simulink model "mahony_alg"  (R2018a)
settings: Solver=FixedStepAuto  StartTime=0.0  StopTime=inf  FixedStep=0.01  RelTol=1e-3  EnableMultiTasking=on
InitFcn:
  | set_param('step_test/Output/Run Sim','Value','1');
  | set_param('step_test/Motor Switch','Value','0');
  | set_param('step_test/Automatic Control','Value','0');
  | %set_param('step_test/Manual PWM','Gain','0');
undefined symbols (not defined in the file or in its folder): sigbuilder_block
libraries: simulink x4, arduinolib x3, dspstat3 x1, dspfdesign x1
settings Model: SimulationMode=external  ExtModeTrigDuration=2  Creator=adiravishankara  LastModifiedBy=adiravishankara
settings SolverCC: AutoInsertRateTranBlk=on
settings OptimizationCC: EnhancedBackFolding=on  PassReuseOutputArgsThreshold=0  MaxStackSize=64  OptimizeBlockOrder=speed  DifferentSizesBufferReuse=on  OptimizationCustomize=off
settings DebuggingCC: ParameterTunabilityLossMsg=error
settings HardwareCC: ProdBitPerPointer=32  ProdBitPerSizeT=32  ProdBitPerPtrDiffT=32  ProdLargestAtomicInteger=Long  ProdLargestAtomicFloat=Double  ProdWordSize=32  ProdHWDeviceType=ARM Compatible->ARM Cortex  UseEmbeddedCoderFeatures=off
settings SFSimCC: MATLABDynamicMemAlloc=off
settings RTWCC: SystemTargetFile=ert.tlc  HardwareBoard=Arduino Due  TLCOptions=-aInlineSetEventsForThisBaseRateFcn=TLC_FALSE -aSuppressMultiTaskScheduler=TLC_FALSE -aRateBasedStepFcn=1  TemplateMakefile=ert_default_tmf  GenerateReport=on  Toolchain=Arduino ARM  BuildConfiguration=Faster Runs  LaunchReport=on
settings CodeAppCC: ForceParamTrailComments=on  OperatorAnnotations=on
settings ERTTargetCC: ERTCustomFileBanners=off  SupportContinuousTime=on  SupportNonInlinedSFcns=on  RemoveResetFunc=off  SupportVariableSizeSignals=on  ModelStepFunctionPrototypeControlCompliant=off

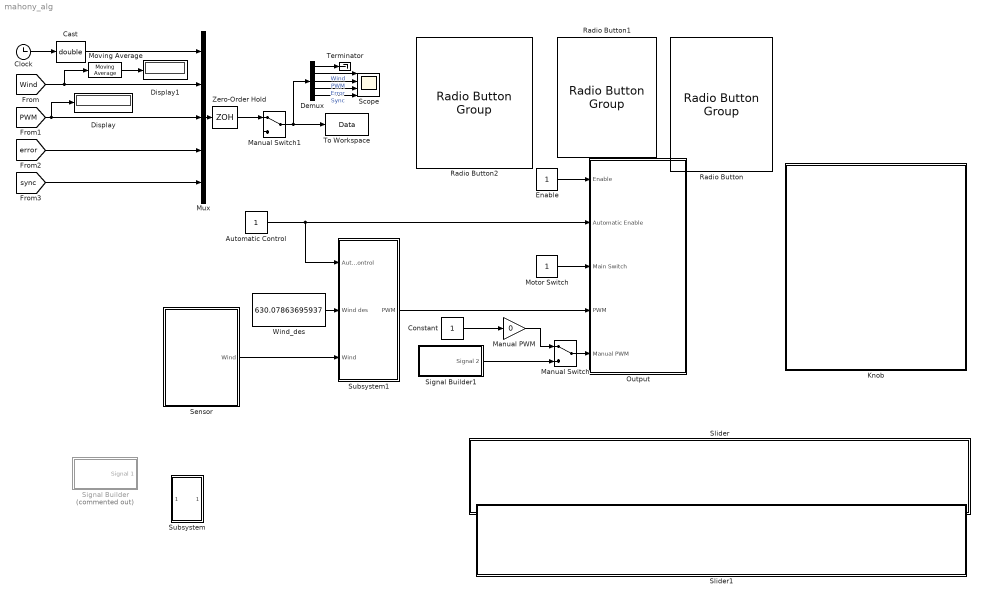
== system mahony_alg ==
  Automatic Control : Constant  SampleTime=0.01
  Cast : DataTypeConversion  OutDataTypeStr=double
  Clock : Clock
  Constant : Constant  SampleTime=0.01
  Demux : Demux  Outputs=5
  Display : Display
  Display1 : Display
  Enable : Constant  SampleTime=0.01
  Knob : Subsystem  DialogController=hmiCreateDDGDialog  IsWebBlock=on  mask(MWDashboardBlock){webBlockId=852d3d9e-f600-4180-8955-96c4171a0510, webBlockType=continuousknob, ShowInLibBrowser=on, ShowInitialText=on, HMISrcModelName=mahony_alg}
      mask prompts: webBlockId "WebBlock Id"; webBlockType "WebBlock Type"; HMISrcModelName "Source Model"
      mask help: SimulinkHMI:dialogs:ContinuousKnobDialogDesc
      mask Help: helpview([docroot '/mapfiles/simulink.map'], 'hmi_knob')
      mask Display:
      | if strcmp(get_param(bdroot(gcb),'BlockDiagramType'), 'library')
      |     image([(matlabroot) '/toolbox/simulink/hmi/icons/ContinuousKnob.png']);
      | end
  Manual PWM : Gain  Gain=0
  Manual Switch : ManualSwitch
  Manual Switch1 : ManualSwitch
  Motor Switch : Constant  SampleTime=0.01
  Moving Average : dspstat3/Moving Average  Method=Sliding window  ForgettingFactorPort=off  SpecifyWindowLength=on  WindowLength=5  ForgettingFactor=0.9  SimulateUsing=Code generation
  Mux : Mux  Inputs=5
  Output : Subsystem
  Radio Button : RadioButtonGroup  WebBlockId=124  SelectedLabel=OFF  ButtonGroupName=SIM STATUS
      settings: Values={{'ON', 'OFF'}, [1 0]}
  Radio Button1 : RadioButtonGroup  WebBlockId=141  SelectedLabel=ON  ButtonGroupName=SIM STATUS
      settings: Values={{'ON', 'OFF'}, [1 0]}
  Radio Button2 : RadioButtonGroup  WebBlockId=144  SelectedLabel=ON  ButtonGroupName=SIM STATUS
      settings: Values={{'ON', 'OFF'}, [1 0]}
  Scope : Scope  NumInputPorts=4
  Sensor : Subsystem
  Signal Builder : Subsystem  Tag=STV Subsys  Commented=on  LoadFcn=sigbuilder_block('load');  StartFcn=sigbuilder_block('start');  StopFcn=sigbuilder_block('stop');  ClipboardFcn=sigbuilder_block('clipboard');  mask(Sigbuilder block){tuvar=[0:10]}
      mask help: Simulink:masks:SigbuilderBlock_MD
      mask init:
      | if ~strcmp(get_param(bdroot(gcbh),'SimulationStatus'),'stopped') tuvar = sigbuilder_block('maskInit'); end
      settings: CopyFcn=sigbuilder_block('copy');  DeleteFcn=sigbuilder_block('delete');  ModelCloseFcn=sigbuilder_block('modelClose');  PreSaveFcn=sigbuilder_block('preSave');  PauseFcn=sigbuilder_block('pause');  ContinueFcn=sigbuilder_block('continue');  NameChangeFcn=sigbuilder_block('namechange');  OpenFcn=sigbuilder_block('open',[48.75 0 1391.25 729.75 ]);  CloseFcn=sigbuilder_block('close');
      mask Display: plot(0, 0, 100, 100,[2, 2, 32, 32, 2], [68, 8, 8, 68, 68],[32, 2], [38, 38], [32, 19, 2],[53, 60, 44], [32, 17, 17, 2],[16, 16, 31, 31]);txt = getActiveGroup(gcbh);text(2, 100, txt,'verticalAlignment', 'top');
  Signal Builder1 : Subsystem  Tag=STV Subsys  LoadFcn=sigbuilder_block('load');  StartFcn=sigbuilder_block('start');  StopFcn=sigbuilder_block('stop');  ClipboardFcn=sigbuilder_block('clipboard');  mask(Sigbuilder block){tuvar=[0:10]}
      mask help: Simulink:masks:SigbuilderBlock_MD
      mask init:
      | if ~strcmp(get_param(bdroot(gcbh),'SimulationStatus'),'stopped') tuvar = sigbuilder_block('maskInit'); end
      settings: CopyFcn=sigbuilder_block('copy');  DeleteFcn=sigbuilder_block('delete');  ModelCloseFcn=sigbuilder_block('modelClose');  PreSaveFcn=sigbuilder_block('preSave');  PauseFcn=sigbuilder_block('pause');  ContinueFcn=sigbuilder_block('continue');  NameChangeFcn=sigbuilder_block('namechange');  OpenFcn=sigbuilder_block('open',[48.75 0 1391.25 711 ]);  CloseFcn=sigbuilder_block('close');
      mask Display: plot(0, 0, 100, 100,[2, 2, 32, 32, 2], [68, 8, 8, 68, 68],[32, 2], [38, 38], [32, 19, 2],[53, 60, 44], [32, 17, 17, 2],[16, 16, 31, 31]);txt = getActiveGroup(gcbh);text(2, 100, txt,'verticalAlignment', 'top');
  Slider : Subsystem  DialogController=hmiCreateDDGDialog  IsWebBlock=on  mask(MWDashboardBlock){webBlockId=6d6bce73-9061-4720-a103-f9820fa904f8, webBlockType=slider, ShowInLibBrowser=on, ShowInitialText=on, HMISrcModelName=mahony_alg}
      mask prompts: webBlockId "WebBlock Id"; webBlockType "WebBlock Type"; HMISrcModelName "Source Model"
      mask help: SimulinkHMI:dialogs:SliderDialogDesc
      mask Help: helpview([docroot '/mapfiles/simulink.map'], 'hmi_slider')
      mask Display:
      | if strcmp(get_param(bdroot(gcb),'BlockDiagramType'), 'library')
      |     image([(matlabroot) '/toolbox/simulink/hmi/icons/Slider.png']);
      | end
  Slider1 : Subsystem  DialogController=hmiCreateDDGDialog  IsWebBlock=on  mask(MWDashboardBlock){webBlockId=583235cf-a666-476d-a93b-c374fcd1b609, webBlockType=slider, ShowInLibBrowser=on, ShowInitialText=on, HMISrcModelName=mahony_alg}
      mask prompts: webBlockId "WebBlock Id"; webBlockType "WebBlock Type"; HMISrcModelName "Source Model"
      mask help: SimulinkHMI:dialogs:SliderDialogDesc
      mask Help: helpview([docroot '/mapfiles/simulink.map'], 'hmi_slider')
      mask Display:
      | if strcmp(get_param(bdroot(gcb),'BlockDiagramType'), 'library')
      |     image([(matlabroot) '/toolbox/simulink/hmi/icons/Slider.png']);
      | end
  Subsystem : Subsystem
  Subsystem1 : Subsystem
  Terminator : Terminator
  To Workspace : ToWorkspace  VariableName=Data  SampleTime=-1
      settings: Save2DSignal=2-D array (concatenate along first dimension)
  Wind_des : Constant  Value=630.07863695937  SampleTime=0.01
  Zero-Order Hold : ZeroOrderHold  SampleTime=0.01
  wires:
  Manual PWM/1 -> Manual Switch/1
  Motor Switch/1 -> Output/3(Main Switch)
  Enable/1 -> Output/1(Enable)
  Constant/1 -> Manual PWM/1
  Wind_des/1 -> Subsystem1/2(Wind des)
  Subsystem1/1(PWM) -> Output/4(PWM)
  Automatic Control/1 -> Subsystem1/1(Automatic Control), Output/2(Automatic Enable)
  Sensor/1(Wind) -> Subsystem1/3(Wind)
  Mux/1 -> Zero-Order Hold/1
  [Wind] -> Mux/2, Moving Average/1
  [PWM] -> Mux/3, Display/1
  [error] -> Mux/4
  Clock/1 -> Cast/1
  Cast/1 -> Mux/1
  [sync] -> Mux/5
  Manual Switch/1 -> Output/5(Manual PWM)
  Moving Average/1 -> Display1/1
  Signal Builder1/1(Signal 2) -> Manual Switch/2
  Manual Switch1/1 -> Demux/1, To Workspace/1
  Zero-Order Hold/1 -> Manual Switch1/1
  Demux/2 -> Scope/1  "Wind"
  Demux/5 -> Scope/4  "Sync"
  Demux/4 -> Scope/3  "Error"
  Demux/3 -> Scope/2  "PWM"
  Demux/1 -> Terminator/1

== system mahony_alg/Knob ==

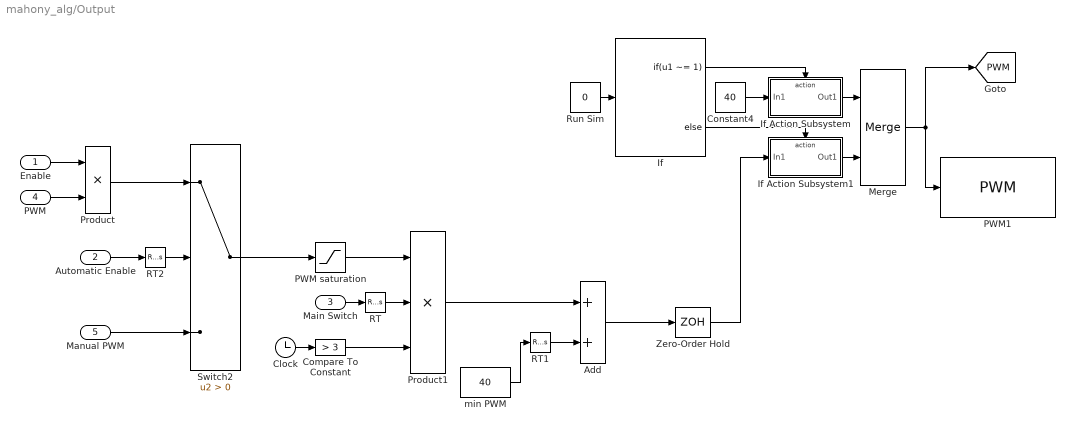
== system mahony_alg/Output ==
  Enable : Inport
  Automatic Enable : Inport  Port=2
  Main Switch : Inport  Port=3
  PWM : Inport  Port=4
  Manual PWM : Inport  Port=5
  Add : Sum
  Clock : Clock
      settings: Decimation=2
  Compare To Constant : simulink/Logic and Bit Operations/Compare To Constant  relop=>  const=3  OutDataTypeStr=boolean
  Constant4 : Constant  Value=40  SampleTime=0.01
  If : If  IfExpression=u1 ~= 1
  If Action Subsystem : Subsystem  TreatAsAtomicUnit=on
  If Action Subsystem1 : Subsystem  TreatAsAtomicUnit=on
  Merge : Merge
  PWM saturation : Saturate  UpperLimit=40  LowerLimit=0
  PWM1 : arduinolib/PWM  pinNumber=12  EnableInputFrequency=off  InitialFrequency=2000  InitialDutyCycle=0  NotificationType=None  blockPlatform=arduino
  Product : Product
  Product1 : Product  Inputs=3
  RT : RateTransition  OutPortSampleTime=0.01
  RT1 : RateTransition  OutPortSampleTime=0.01
  RT2 : RateTransition  OutPortSampleTime=0.01
  Run Sim : Constant  Value=0  SampleTime=0.01
  Switch2 : Switch  Criteria=u2 > Threshold
  Zero-Order Hold : ZeroOrderHold  SampleTime=0.01
  min PWM : Constant  Value=40  SampleTime=0.01
  tag scope: PWM=global
  wires:
  Clock/1 -> Compare To Constant/1
  min PWM/1 -> RT1/1
  Compare To Constant/1 -> Product1/3
  Automatic Enable/1 -> RT2/1
  Manual PWM/1 -> Switch2/3
  PWM/1 -> Product/2
  Switch2/1 -> PWM saturation/1
  Main Switch/1 -> RT/1
  Product1/1 -> Add/1
  PWM saturation/1 -> Product1/1
  Product/1 -> Switch2/1
  Enable/1 -> Product/1
  If/1 -> If Action Subsystem/Action
  Run Sim/1 -> If/1
  Constant4/1 -> If Action Subsystem/1(In1)
  Add/1 -> Zero-Order Hold/1
  If/2 -> If Action Subsystem1/Action
  If Action Subsystem/1(Out1) -> Merge/1
  If Action Subsystem1/1(Out1) -> Merge/2
  Merge/1 -> PWM1/1, [PWM]
  Zero-Order Hold/1 -> If Action Subsystem1/1(In1)
  RT/1 -> Product1/2
  RT1/1 -> Add/2
  RT2/1 -> Switch2/2

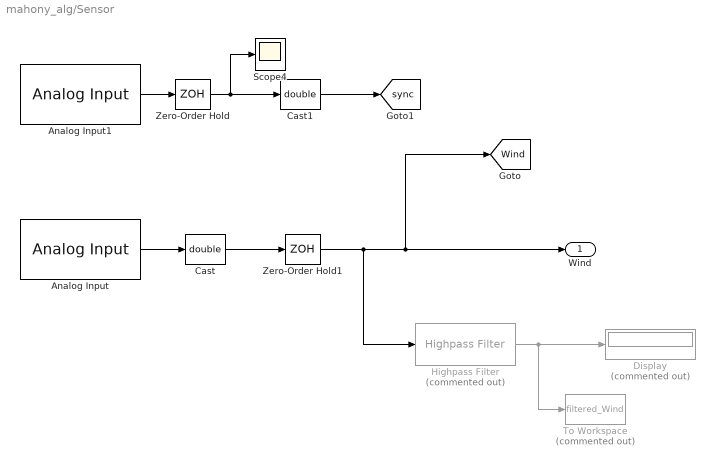
== system mahony_alg/Sensor ==
  Analog Input : arduinolib/Analog Input  pinNumber=2  ReadResultsOnly=off  ConversionTriggerSource=Software  ExternalTriggerType=uint32(0)  OutputDataType=uint16  EnableConversionCompleteNotify=off  EnableOuputStatus=off  SampleTime=0.01  blockPlatform=arduino
  Analog Input1 : arduinolib/Analog Input  pinNumber=3  ReadResultsOnly=off  ConversionTriggerSource=Software  ExternalTriggerType=uint32(0)  OutputDataType=uint16  EnableConversionCompleteNotify=off  EnableOuputStatus=off  SampleTime=0.01  blockPlatform=arduino
  Cast : DataTypeConversion  OutDataTypeStr=double
  Cast1 : DataTypeConversion  OutDataTypeStr=double
  Display : Display  Commented=on
  Highpass Filter : dspfdesign/Highpass Filter  Commented=on  FilterType=FIR  DesignForMinimumOrder=on  FilterOrder=50  StopbandFrequency=8e3  PassbandFrequency=12e3  StopbandAttenuation=80  PassbandRipple=0.1  InheritSampleRate=on  SampleRate=44100  SimulateUsing=Interpreted execution  roundingMode=Floor  coeffsDataTypeStr=fixdt(1,16)
      settings: SourceProductName=DSP System Toolbox
  Scope4 : Scope
  To Workspace : ToWorkspace  Commented=on  VariableName=filtered_Wind  SampleTime=0.01
  Zero-Order Hold : ZeroOrderHold  SampleTime=0.01
  Zero-Order Hold1 : ZeroOrderHold  SampleTime=0.01
  Wind : Outport
  tag scope: Wind=global, sync=global
  wires:
  Zero-Order Hold/1 -> Cast1/1, Scope4/1
  Analog Input/1 -> Cast/1
  Cast/1 -> Zero-Order Hold1/1
  Analog Input1/1 -> Zero-Order Hold/1
  Cast1/1 -> [sync]
  Zero-Order Hold1/1 -> Highpass Filter/1, Wind/1, [Wind]
  Highpass Filter/1 -> To Workspace/1, Display/1

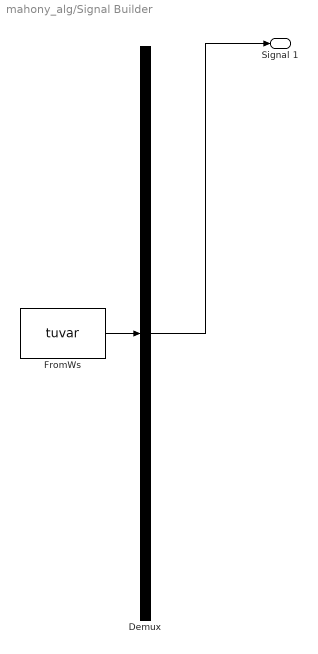
== system mahony_alg/Signal Builder ==
  Demux : Demux  Tag=STV Demux  Outputs=1
  FromWs : FromWorkspace  Tag=STV FromWs  VariableName=tuvar  SampleTime=0
      SigBuilderData=|
      | common.afterFinalStr = 'Extrapolate'
      | common.sampleTime = 0
      | dataSet.timeRange = [0 500]
      | dataSet.name = 'Group 1'
      | sbobj.Groups.Name = 'Group 1'
      | sbobj.Groups.Signals.Name = 'Signal 1'
      | sbobj.Groups.Signals.XData = [0 10 10 30 30 50 50 70 70 90 90 110 110 130 130 150 150 170 170 190 190 210 210 230 230 250 250 270 270 289 290 310 310 330 330 350 350 370 370 390 390 410 410 450 450 500]
      | sbobj.Groups.Signals.YData = [0 0 4 4 4.1 4.1 4.2 4.2 4.3 4.3 4.4 4.4 4.5 4.5 4.6 4.6 4.7 4.7 4.8 4.8 4.9 4.9 5 5 5.1 5.1 5.2 5.2 5.3 5.3 5.4 5.4 5.5 5.5 5.6 5.6 5.7 5.7 5.8 5.8 5.9 5.9 6 6 0 0]
      | sbobj.Groups.TimeRange = [0 500]
  Signal 1 : Outport  Tag=STV Outport
  wires:
  Demux/1 -> Signal 1/1
  FromWs/1 -> Demux/1

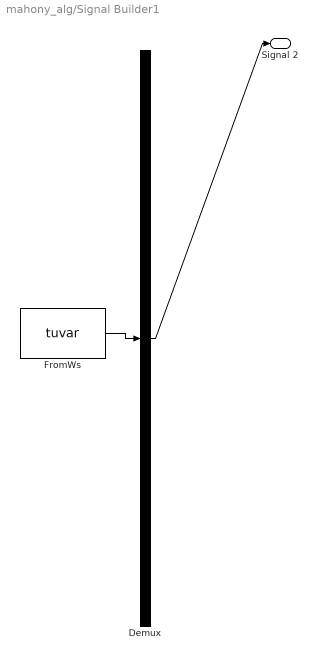
== system mahony_alg/Signal Builder1 ==
  Demux : Demux  Tag=STV Demux  Outputs=1
  FromWs : FromWorkspace  Tag=STV FromWs  VariableName=tuvar  SampleTime=0
      SigBuilderData=|
      | common.afterFinalStr = 'Extrapolate'
      | common.sampleTime = 0
      | dataSet.timeRange = [0 300]
      | dataSet.name = 'Group 1'
      | sbobj.Groups.Name = 'Group 1'
      | sbobj.Groups.Signals.Name = 'Signal 2'
      | sbobj.Groups.Signals.XData = [0 60 60 119 119 179 179 239 239 299 299 300]
      | sbobj.Groups.Signals.YData = [0 0 4 4 5 5 6 6 7 7 8 8]
      | sbobj.Groups.TimeRange = [0 300]
  Signal 2 : Outport  Tag=STV Outport
  wires:
  FromWs/1 -> Demux/1
  Demux/1 -> Signal 2/1

== system mahony_alg/Slider ==

== system mahony_alg/Slider1 ==

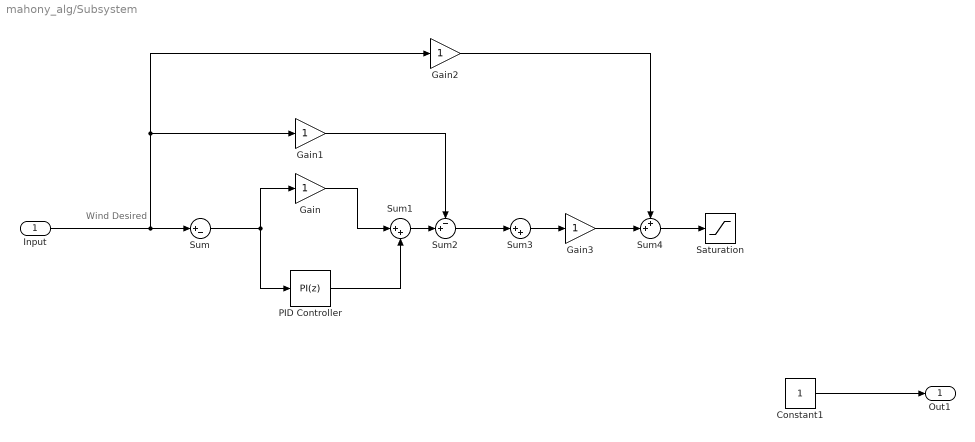
== system mahony_alg/Subsystem ==
  note: Wind Desired
  Input : Inport
  Constant1 : Constant
  Gain{,1..3} (4 alike) : Gain
  PID Controller : simulink/Continuous/PID Controller  Controller=PI  TimeDomain=Discrete-time  SampleTime=-1  IntegratorMethod=Forward Euler  FilterMethod=Forward Euler  Form=Parallel  UseFilter=on  ControllerParametersSource=internal  P=1  I=1  D=0  N=100  InitialConditionSource=internal  InitialConditionForIntegrator=0  InitialConditionForFilter=0  ExternalReset=none  LimitOutput=off  UpperSaturationLimit=inf  LowerSaturationLimit=-inf  LinearizeAsGain=on  AntiWindupMode=none  Kb=1  TrackingMode=off  Kt=1  PParamMin=[]  PParamMax=[]  IParamMin=[]  IParamMax=[]  DParamMin=[]  DParamMax=[]  NParamMin=[]  NParamMax=[]  KbParamMin=[]  KbParamMax=[]  KtParamMin=[]  KtParamMax=[]  POutMin=[]  POutMax=[]  IOutMin=[]  IOutMax=[]  DOutMin=[]  DOutMax=[]  NOutMin=[]  NOutMax=[]  KbOutMin=[]  KbOutMax=[]  KtOutMin=[]  KtOutMax=[]  IntegratorOutMin=[]  IntegratorOutMax=[]  FilterOutMin=[]  FilterOutMax=[]  SumOutMin=[]  SumOutMax=[]  SumI1OutMin=[]  SumI1OutMax=[]  SumI2OutMin=[]  SumI2OutMax=[]  SumI3OutMin=[]  SumI3OutMax=[]  SumDOutMin=[]  SumDOutMax=[]  SaturationOutMin=[]  SaturationOutMax=[]  IntegratorContinuousStateAttributes=''  IntegratorStateMustResolveToSignalObject=off  IntegratorRTWStateStorageClass=Auto  FilterContinuousStateAttributes=''  FilterStateMustResolveToSignalObject=off  FilterRTWStateStorageClass=Auto  DifferentiatorICPrevScaledInput=0  DifferentiatorOutMin=[]  DifferentiatorOutMax=[]  InitialConditionSetting=Output  FilterDiffOutCoefMin=[]  FilterDiffOutCoefMax=[]  SumDenOutMin=[]  SumDenOutMax=[]  SumNumOutMin=[]  SumNumOutMax=[]  ReciprocalOutMin=[]  ReciprocalOutMax=[]  DivideOutMin=[]  DivideOutMax=[]  TunerSelectOption=Transfer Function Based (PID Tuner App)
  Saturation : Saturate
  Sum : Sum  Inputs=|+-
  Sum1 : Sum  Inputs=|++
  Sum2 : Sum  Inputs=-+|
  Sum3 : Sum  Inputs=|++
  Sum4 : Sum  Inputs=++|
  Out1 : Outport
  wires:
  Constant1/1 -> Out1/1
  Input/1 -> Sum/1, Gain2/1, Gain1/1
  Sum/1 -> PID Controller/1, Gain/1
  Gain/1 -> Sum1/1
  PID Controller/1 -> Sum1/2
  Sum1/1 -> Sum2/2
  Gain1/1 -> Sum2/1
  Sum2/1 -> Sum3/1
  Sum3/1 -> Gain3/1
  Gain3/1 -> Sum4/2
  Gain2/1 -> Sum4/1
  Sum4/1 -> Saturation/1

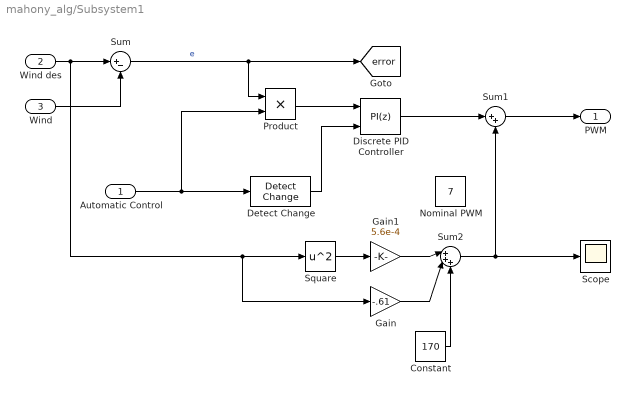
== system mahony_alg/Subsystem1 ==
  Automatic Control : Inport
  Wind des : Inport  Port=2
  Wind : Inport  Port=3
  Constant : Constant  Value=170
  Detect Change : simulink/Logic and Bit Operations/Detect Change  vinit=0  OutDataTypeStr=boolean
  Discrete PID Controller : simulink/Continuous/PID Controller  Controller=PI  TimeDomain=Discrete-time  SampleTime=0.01  IntegratorMethod=Forward Euler  FilterMethod=Forward Euler  Form=Parallel  UseFilter=on  ControllerParametersSource=internal  P=0.05  I=0.01  D=0  N=100  InitialConditionSource=internal  InitialConditionForIntegrator=0  InitialConditionForFilter=0  ExternalReset=rising  LimitOutput=off  UpperSaturationLimit=inf  LowerSaturationLimit=-inf  LinearizeAsGain=off  AntiWindupMode=none  Kb=1  TrackingMode=off  Kt=1  PParamMin=[]  PParamMax=[]  IParamMin=[]  IParamMax=[]  DParamMin=[]  DParamMax=[]  NParamMin=[]  NParamMax=[]  KbParamMin=[]  KbParamMax=[]  KtParamMin=[]  KtParamMax=[]  POutMin=[]  POutMax=[]  IOutMin=[]  IOutMax=[]  DOutMin=[]  DOutMax=[]  NOutMin=[]  NOutMax=[]  KbOutMin=[]  KbOutMax=[]  KtOutMin=[]  KtOutMax=[]  IntegratorOutMin=[]  IntegratorOutMax=[]  FilterOutMin=[]  FilterOutMax=[]  SumOutMin=[]  SumOutMax=[]  SumI1OutMin=[]  SumI1OutMax=[]  SumI2OutMin=[]  SumI2OutMax=[]  SumI3OutMin=[]  SumI3OutMax=[]  SumDOutMin=[]  SumDOutMax=[]  SaturationOutMin=[]  SaturationOutMax=[]  IntegratorContinuousStateAttributes=''  IntegratorStateMustResolveToSignalObject=off  IntegratorRTWStateStorageClass=Auto  FilterContinuousStateAttributes=''  FilterStateMustResolveToSignalObject=off  FilterRTWStateStorageClass=Auto  DifferentiatorICPrevScaledInput=0  DifferentiatorOutMin=[]  DifferentiatorOutMax=[]  FilterDiffOutCoefMin=[]  FilterDiffOutCoefMax=[]  SumDenOutMin=[]  SumDenOutMax=[]  SumNumOutMin=[]  SumNumOutMax=[]  ReciprocalOutMin=[]  ReciprocalOutMax=[]  DivideOutMin=[]  DivideOutMax=[]  TunerSelectOption=Transfer Function Based (PID Tuner App)
  Gain : Gain  Gain=-.61
  Gain1 : Gain  Gain=5.6e-4
  Nominal PWM : Constant  Value=7  SampleTime=0.01
  Product : Product
  Scope : Scope
  Square : Math  Operator=square  SaturateOnIntegerOverflow=on
  Sum : Sum  Inputs=|+-
  Sum1 : Sum  Inputs=|++
  Sum2 : Sum  Inputs=|+++
  PWM : Outport
  tag scope: error=global
  wires:
  Detect Change/1 -> Discrete PID Controller/2
  Wind des/1 -> Gain/1, Square/1, Sum/1
  Discrete PID Controller/1 -> Sum1/1
  Sum/1 -> [error], Product/1  "e"
  Wind/1 -> Sum/2
  Automatic Control/1 -> Product/2, Detect Change/1
  Sum1/1 -> PWM/1
  Product/1 -> Discrete PID Controller/1
  Gain/1 -> Sum2/2
  Gain1/1 -> Sum2/1
  Constant/1 -> Sum2/3
  Square/1 -> Gain1/1
  Sum2/1 -> Sum1/2, Scope/1

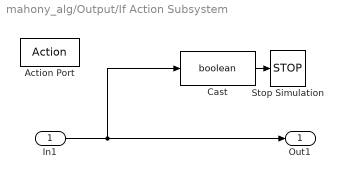
== system mahony_alg/Output/If Action Subsystem ==
  In1 : Inport
  Action Port : ActionPort  ActionType=then
  Cast : DataTypeConversion  OutDataTypeStr=boolean
  Stop Simulation : Stop
  Out1 : Outport
  wires:
  In1/1 -> Cast/1, Out1/1
  Cast/1 -> Stop Simulation/1

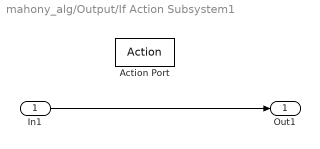
== system mahony_alg/Output/If Action Subsystem1 ==
  In1 : Inport
  Action Port : ActionPort  ActionType=else
  Out1 : Outport
  wires:
  In1/1 -> Out1/1
